simulink model "VFA_lin"  (Simulink 9.0)
settings: Solver=ode45  StartTime=0.0  StopTime=10.0  RelTol=1e-3  EnableMultiTasking=on
undefined symbols (not defined in the file or in its folder): data, stateinit
settings Model: SuppressorTable=22 serialization::archive 11 0 6 0 0 0 0 0  Creator=Travis  LastModifiedBy=ben
settings DataIOCC: LimitDataPoints=on  SignalLoggingSaveFormat=ModelDataLogs
settings OptimizationCC: BlockReduction=off  DefaultParameterBehavior=Inlined  BufferReuse=off  ExpressionDepthLimit=2147483647  InitFltsAndDblsToZero=on
settings DebuggingCC: SaveWithParameterizedLinksMsg=none  SignalResolutionControl=TryResolveAllWithWarning  SolverPrmCheckMsg=warning  MultiTaskDSMMsg=warning  MultiTaskCondExecSysMsg=none  FcnCallInpInsideContextMsg=warning  StateNameClashWarn=warning  InitInArrayFormatMsg=none  StrictBusMsg=Warning
settings GRTTargetCC: TargetFcnLib=ansi_tfl_tmw.mat  GeneratePreprocessorConditionals=Disable all  CombineOutputUpdateFcns=off  GRTInterface=on

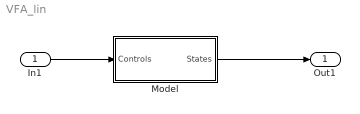
== system VFA_lin ==
  In1 : Inport
  Model : Subsystem
  Out1 : Outport
  wires:
  Model/1(States) -> Out1/1
  In1/1 -> Model/1(Controls)

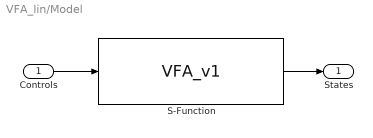
== system VFA_lin/Model ==
  Controls : Inport
  S-Function : S-Function  FunctionName=VFA_v1  Parameters=data,stateinit  SFunctionDeploymentMode=off  EnableBusSupport=off
  States : Outport
  wires:
  Controls/1 -> S-Function/1
  S-Function/1 -> States/1
